simulink model "controllerdesign"  (R2017a)
settings: Solver=VariableStepAuto  StartTime=0.0  StopTime=10.0  RelTol=1e-3
settings Model: Creator=Jash  LastModifiedBy=Jash

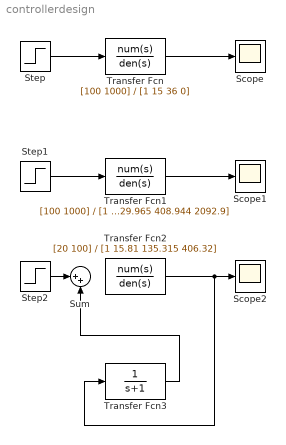
== system controllerdesign ==
  Scope : Scope
  Scope1 : Scope
  Scope2 : Scope
  Step : Step  Time=0  SampleTime=0
  Step1 : Step  Time=0  After=2  SampleTime=0
  Step2 : Step  Time=0  SampleTime=0
  Sum : Sum  Inputs=|++
  Transfer Fcn : TransferFcn  Numerator=[100 1000]  Denominator=[1 15 36 0]
  Transfer Fcn1 : TransferFcn  Numerator=[100 1000]  Denominator=[1 29.965 408.944 2092.9]
  Transfer Fcn2 : TransferFcn  Numerator=[20 100]  Denominator=[1 15.81 135.315 406.32]
  Transfer Fcn3 : TransferFcn  Denominator=[1 1]
  wires:
  Transfer Fcn/1 -> Scope/1
  Step/1 -> Transfer Fcn/1
  Step1/1 -> Transfer Fcn1/1
  Transfer Fcn1/1 -> Scope1/1
  Transfer Fcn2/1 -> Transfer Fcn3/1, Scope2/1
  Step2/1 -> Sum/1
  ? -> Transfer Fcn2/1
  Transfer Fcn3/1 -> Sum/2
